simulink model "Vary_Systemu"  (R2021a)
settings: Solver=VariableStepAuto  StartTime=0.0  StopTime=49000  FixedStep=0.01  RelTol=1e-3
values from neighbouring files (symbols this model uses):
  Ts = 0.5    [Distillation_Column_model_identification.m]    (also in Distillation_Column_model_variance.m; fourvary.m = 8)
libraries: cstblocks x2, pid_lib x1, dspsrcs4 x1, simulink x1
settings Model: Creator=沈远义  LastModifiedBy=dell
settings DataIOCC: LoadExternalInput=on

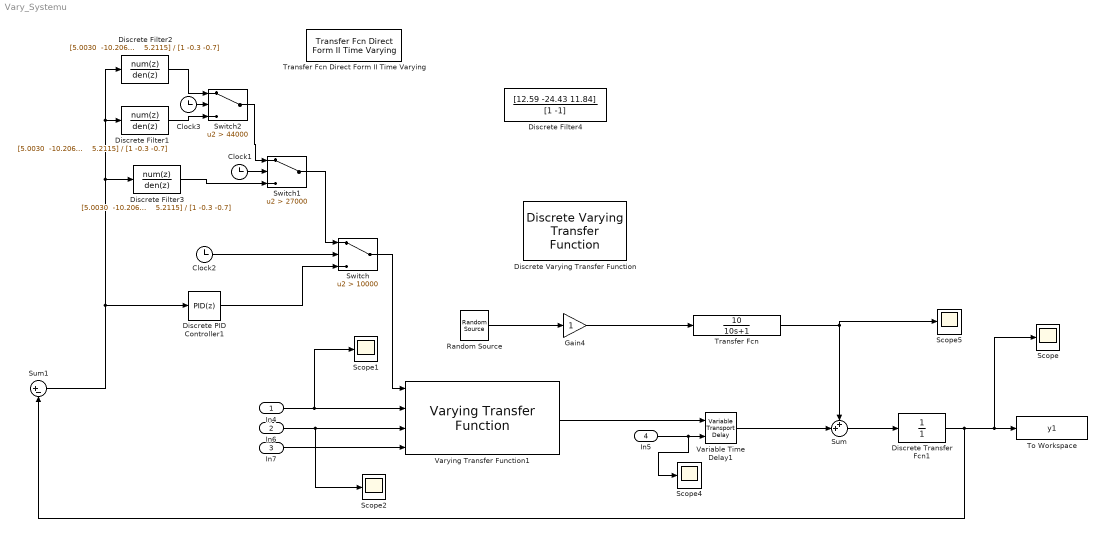
== system Vary_Systemu ==
  In4 : Inport
  In6 : Inport  Port=2
  In7 : Inport  Port=3
  In5 : Inport  Port=4
  Clock1 : Clock
  Clock2 : Clock
  Clock3 : Clock
  Discrete Transfer Fcn1 : DiscreteTransferFcn  Denominator=[1]  SampleTime=Ts
  Discrete Filter1 : DiscreteFilter  Numerator="[5.0030  -10.2067    5.2115]"  Denominator=[1 -0.3 -0.7]
  Discrete Filter2 : DiscreteFilter  Numerator="[5.0030  -10.2067    5.2115]"  Denominator=[1 -0.3 -0.7]
  Discrete Filter3 : DiscreteFilter  Numerator="[5.0030  -10.2067    5.2115]"  Denominator=[1 -0.3 -0.7]
  Discrete Filter4 : DiscreteFilter  Numerator=[12.59 -24.43 11.84]  Denominator=[1 -1]
  Discrete PID Controller1 : pid_lib/PID Controller  Controller=PID  Form=Parallel  TimeDomain=Discrete-time  UseExternalTs=off  SampleTime=-1  IntegratorMethod=Forward Euler  FilterMethod=Forward Euler  ControllerParametersSource=internal  P=0.745875669585536  I=0.00622991619120585  D=11.8431061933714  UseFilter=off  N=100  TunerSelectOption=Transfer Function Based (PID Tuner App)  InitialConditionSource=internal  InitialConditionForIntegrator=0  InitialConditionForFilter=0  DifferentiatorICPrevScaledInput=0  ExternalReset=none  TrackingMode=off  Kt=1  LimitOutput=off  SatLimitsSource=internal  UpperSaturationLimit=inf  LowerSaturationLimit=-inf  LinearizeAsGain=off  AntiWindupMode=none  Kb=1  POutMin=[]  POutMax=[]  IOutMin=[]  IOutMax=[]  DOutMin=[]  DOutMax=[]  NOutMin=[]  NOutMax=[]  SumOutMin=[]  SumOutMax=[]  SaturationOutMin=[]  SaturationOutMax=[]  PParamMin=[]  PParamMax=[]  IParamMin=[]  IParamMax=[]  DParamMin=[]  DParamMax=[]  NParamMin=[]  NParamMax=[]  KbParamMin=[]  KbParamMax=[]  KtParamMin=[]  KtParamMax=[]  KbOutMin=[]  KbOutMax=[]  KtOutMin=[]  KtOutMax=[]  IntegratorOutMin=[]  IntegratorOutMax=[]  FilterOutMin=[]  FilterOutMax=[]  SumI1OutMin=[]  SumI1OutMax=[]  SumI2OutMin=[]  SumI2OutMax=[]  SumI3OutMin=[]  SumI3OutMax=[]  SumI4OutMin=[]  SumI4OutMax=[]  SumDOutMin=[]  SumDOutMax=[]  DifferentiatorOutMin=[]  DifferentiatorOutMax=[]  FilterDiffOutCoefMin=[]  FilterDiffOutCoefMax=[]  ReciprocalOutMin=[]  ReciprocalOutMax=[]  SumDenOutMin=[]  SumDenOutMax=[]  SumNumOutMin=[]  SumNumOutMax=[]  DivideOutMin=[]  DivideOutMax=[]  UdiffTsProdOutMin=[]  UdiffTsProdOutMax=[]  NTsProdOutMin=[]  NTsProdOutMax=[]  UintegralTsProdOutMin=[]  UintegralTsProdOutMax=[]  UngainTsProdOutMin=[]  UngainTsProdOutMax=[]  IntegratorContinuousStateAttributes=''  IntegratorStateMustResolveToSignalObject=off  IntegratorRTWStateStorageClass=Auto  FilterContinuousStateAttributes=''  FilterStateMustResolveToSignalObject=off  FilterRTWStateStorageClass=Auto  ParallelPVariant=InternalParameters  IdealPVariant=Disabled  IVariant=InternalParameters  DVariant=InternalParameters  IntegratorVariant=Discrete  SatVariant=Disabled  AWVariant=Passthrough  PCopyVariant=Disabled  TRVariant=Disabled  FdbkBlocksVariant=Forward  IdealPFdbkVariant=Disabled  SatFdbkVariant=Disabled  DerivativeFilterVariant=Differentiator  NVariant=Passthrough  NCopyVariant=Disabled_SignalSpec  FilterICVariant=InternalICsDifferentiator  IntegratorICVariant=InternalICs  ExternalResetVariant=Disabled  TRSumVariant=Passthrough  SumFdbkVariant=Disabled  SumVariant=Sum_PID  TsampFilterVariant=InternalTs  TsampNgainVariant=Passthrough  TsampIntegralVariant=Passthrough  ExternalSaturationOutDataTypeStr=Inherit: Same as second input
  Discrete Varying Transfer Function : cstblocks/Linear Parameter Varying/Discrete Varying Transfer Function  N=3  Ts=-1
      settings: SourceProductBaseCode=CT
  Gain4 : Gain
  Random Source : dspsrcs4/Random Source  SrcType=Gaussian  NormMethod=Ziggurat  CltLength=12  MinVal=-1  MaxVal=1  MeanVal=0  VarVal=1  RepMode=Specify seed  rawSeed=1  IsInherit=off  SampMode=Continuous  SampTime=1  SampFrame=1  DataType=Double  OutComplex=Real  OutputFrames=off
  Scope{,1..2,4..5} (5 alike) : Scope
  Sum : Sum  Inputs=++|
  Sum1 : Sum  Inputs=|+-
  Switch : Switch  Criteria=u2 > Threshold  Threshold=10000
  Switch1 : Switch  Criteria=u2 > Threshold  Threshold=27000
  Switch2 : Switch  Criteria=u2 > Threshold  Threshold=44000
  To Workspace : ToWorkspace  VariableName=y1  SampleTime=-1
  Transfer Fcn : TransferFcn  Numerator=[10]  Denominator=[10 1]
  Transfer Fcn Direct Form II Time Varying : simulink/Additional Math & Discrete/Additional Discrete/Transfer Fcn Direct Form II Time Varying  vinit=0.0  DoSatur=off
      settings: SourceProductBaseCode=SL
  Variable Time Delay1 : VariableTransportDelay  MaximumDelay=200
  Varying Transfer Function1 : cstblocks/Linear Parameter Varying/Varying Transfer Function  N=1
  wires:
  In5/1 -> Scope4/1, Variable Time Delay1/2
  In6/1 -> Scope2/1, Varying Transfer Function1/3
  In4/1 -> Scope1/1, Varying Transfer Function1/2
  In7/1 -> Varying Transfer Function1/4
  Varying Transfer Function1/1 -> Variable Time Delay1/1
  Variable Time Delay1/1 -> Sum/2
  Random Source/1 -> Gain4/1
  Sum/1 -> Discrete Transfer Fcn1/1
  Discrete Transfer Fcn1/1 -> Scope/1, To Workspace/1, Sum1/2
  Clock2/1 -> Switch/2
  Discrete PID Controller1/1 -> Switch/3
  Switch/1 -> Varying Transfer Function1/1
  Switch1/1 -> Switch/1
  Clock1/1 -> Switch1/2
  Clock3/1 -> Switch2/2
  Switch2/1 -> Switch1/1
  Discrete Filter1/1 -> Switch2/3
  Gain4/1 -> Transfer Fcn/1
  Transfer Fcn/1 -> Sum/1, Scope5/1
  Discrete Filter2/1 -> Switch2/1
  Sum1/1 -> Discrete PID Controller1/1, Discrete Filter3/1, Discrete Filter2/1, Discrete Filter1/1
  Discrete Filter3/1 -> Switch1/3
